simulink model "plausability_control_simulink"  (R2020b)
settings: Solver=VariableStepAuto  StartTime=0.0  StopTime=10.0  RelTol=1e-3
libraries: simulink x3
settings Model: Creator=dobos  LastModifiedBy=dobos

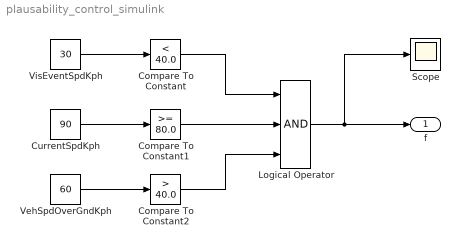
== system plausability_control_simulink ==
  " VehSpdOverGndKph" : Constant  Value=60
  Compare To Constant : simulink/Logic and Bit Operations/Compare To Constant  relop=<  const=40.0  OutDataTypeStr=boolean
  Compare To Constant1 : simulink/Logic and Bit Operations/Compare To Constant  relop=>=  const=80.0  OutDataTypeStr=boolean
  Compare To Constant2 : simulink/Logic and Bit Operations/Compare To Constant  relop=>  const=40.0  OutDataTypeStr=boolean
  CurrentSpdKph : Constant  Value=90
  Logical Operator : Logic  Inputs=3  AllPortsSameDT=off  OutDataTypeStr=boolean
  Scope : Scope
  VisEventSpdKph : Constant  Value=30
  f : Outport
  wires:
  " VehSpdOverGndKph"/1 -> Compare To Constant2/1
  CurrentSpdKph/1 -> Compare To Constant1/1
  VisEventSpdKph/1 -> Compare To Constant/1
  Compare To Constant/1 -> Logical Operator/1
  Compare To Constant1/1 -> Logical Operator/2
  Compare To Constant2/1 -> Logical Operator/3
  Logical Operator/1 -> f/1, Scope/1
